simulink model "RCAM_script_sim"  (R2023a)
settings: Solver=VariableStepAuto  StartTime=0.0  StopTime=TF  RelTol=1e-3
values from neighbouring files (symbols this model uses):
  u0 = [0 ... (first row only)    [RCAM_script_run.m]
  x0 = [85 ... (first row only)    [RCAM_script_run.m]
undefined symbols (not defined in the file or in its folder): RCAM_script_dynamics
settings Model: Creator=Reggie Johanes  LastModifiedBy=Reggie Johanes

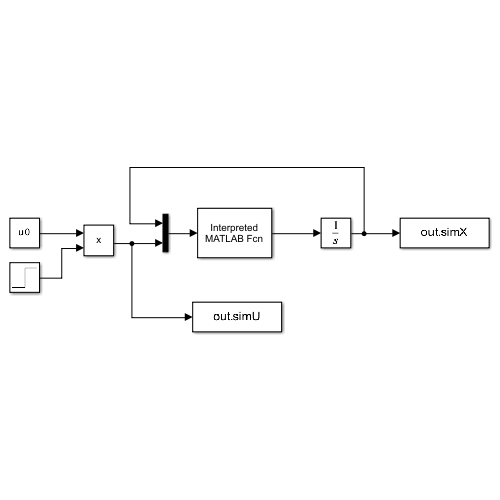
[thumbnail: Simulink's stored preview of the top-level diagram]
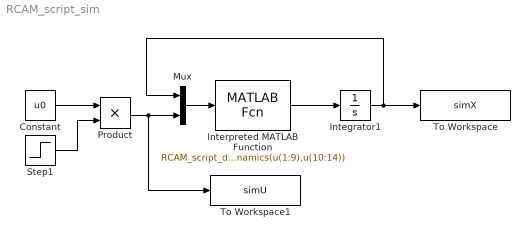
== system RCAM_script_sim ==
  Constant : Constant  Value=u0
  Integrator1 : Integrator  InitialCondition=x0
  Interpreted MATLAB Function : MATLABFcn  MATLABFcn=RCAM_script_dynamics(u(1:9),u(10:14))
  Mux : Mux  Inputs=2
  Product : Product
  Step1 : Step  Time=0  SampleTime=0
  To Workspace : ToWorkspace  VariableName=simX  SaveFormat=Timeseries  SampleTime=-1
  To Workspace1 : ToWorkspace  VariableName=simU  SaveFormat=Timeseries  SampleTime=-1
  wires:
  Mux/1 -> Interpreted MATLAB Function/1
  Integrator1/1 -> To Workspace/1, Mux/1
  Interpreted MATLAB Function/1 -> Integrator1/1
  Constant/1 -> Product/1
  Step1/1 -> Product/2
  Product/1 -> Mux/2, To Workspace1/1
